simulink model "two_tanks"  (R2013b)
settings: Solver=ode45  SolverMode=SingleTasking  StartTime=0.0  StopTime=10  RelTol=1e-3
settings Model: Creator=The MathWorks Inc.  LastModifiedBy=Daniel
settings DataIOCC: SignalLoggingSaveFormat=ModelDataLogs
settings OptimizationCC: BlockReduction=off  BooleanDataType=off  ExpressionDepthLimit=2147483647  InitFltsAndDblsToZero=on
settings DebuggingCC: SignalResolutionControl=TryResolveAllWithWarning  SolverPrmCheckMsg=none  FcnCallInpInsideContextMsg=UseLocalSettings  StateNameClashWarn=warning
settings HardwareCC: TargetUnknown=on
settings SFSimCC: SFSimEnableDebug=off  SFSimOverflowDetection=off  SFSimEcho=off  SimParseCustomCode=off
settings GRTTargetCC: TargetFcnLib=ansi_tfl_tmw_new.mat  CombineOutputUpdateFcns=off  GRTInterface=on

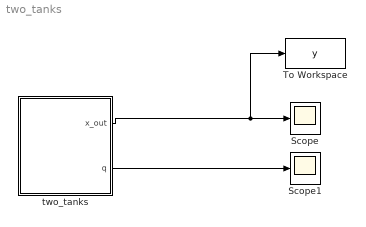
== system two_tanks ==
  Scope : Scope
      settings: YMin=-0.75  YMax=0.75
  Scope1 : Scope
      settings: YMin=-0.75  YMax=0.75
  To Workspace : ToWorkspace  VariableName=y  SampleTime=-1
  two_tanks : Stateflow chart  TreatAsAtomicUnit=on
  wires:
  two_tanks/1(x_out) -> Scope/1, To Workspace/1
  two_tanks/2(q) -> Scope1/1

== stateflow chart two_tanks/two_tanks ==
  settings: updateMethod=CONTINUOUS  executeAtInitialization=1  initializeOutput=1
  state Filling_Tank_1
    du:
    q = 1;
    x_out = x;
    x_dot[0] = w-v[0];
    x_dot[1] = -v[1];
  state Filling_Tank_2
    du:
    q = 2;
    x_out = x;
    x_dot[0] = -v[0];
    x_dot[1] = w-v[1];
  (default) -> Filling_Tank_1 : {
      | x[0] = 5;
      | x[1] = 4;
      | }
  Filling_Tank_2 -> Filling_Tank_1 : [ x[0] < r[0] ]
  Filling_Tank_1 -> Filling_Tank_2 : [ x[1] < r[1] ]
  data: x_out output double size=2; w constant double =5; r constant double size=2 =[2 1]; x local double size=2; v constant double size=2 =[3 2]; q output double
  data x settings: updateMethod=SF_CONTINUOUS_TIME_DATA
